simulink model "MCSI_simulation_2024_final_sim"  (R2021a)
settings: Solver=VariableStepAuto  StartTime=0.0  StopTime=10/cfg.fl  RelTol=1e-3
undefined symbols (not defined in the file or in its folder): cfg
libraries: spsIdealSwitchLib x18, simulink x17, hdlsllib x12, spsSeriesRLCBranchLib x8, spsCurrentMeasurementLib x6, commutil2 x6, spsMosfetLib x4, spsTriangleGeneratorLib x3, spsThreePhaseProgrammableGeneratorLib x3, spsMeanLib x2, spsThreePhaseSeriesRLCBranchLib x2, spsThreePhaseVIMeasurementLib x2
(part 1 of 2)
settings Model: Creator=Damian  LastModifiedBy=Damian

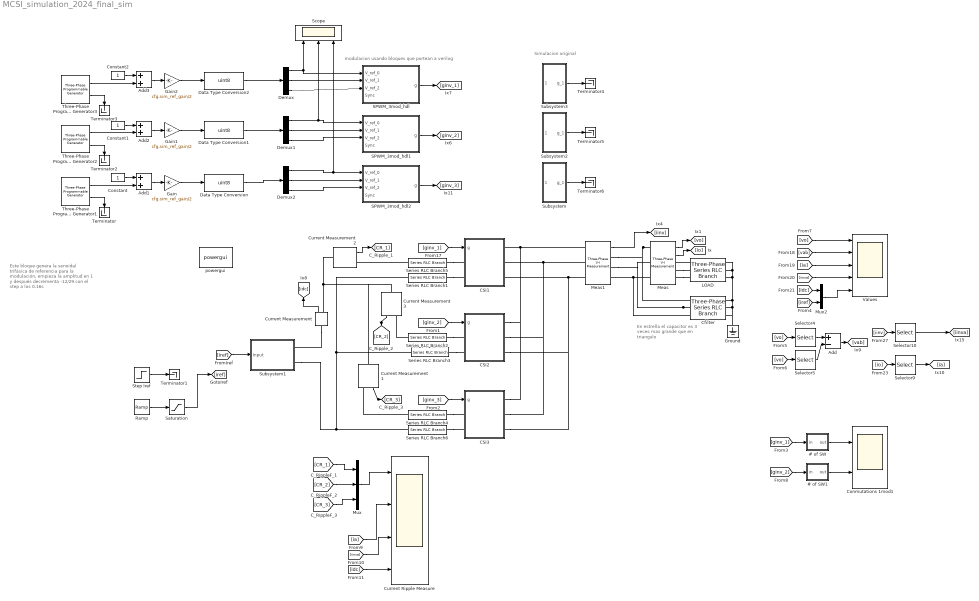
== system MCSI_simulation_2024_final_sim ==
  note: modulacion usando bloques que portean a verilog
  note: Simulacion original
  note: Este bloque genera la senoidal
      | trifásica de referencia para la
      | modulación, empieza la amplitud
      | en 1 y después decrementa -12/29
      | con el step a los 0.16s
  note: En estrella el capacitor
      | es 3 veces mas grande
      | que en triangulo
  # of SW : Subsystem
  # of SW1 : Subsystem
  Add : Sum  Inputs=+-
  Add1 : Sum
  Add2 : Sum
  Add3 : Sum
  CSI1 : Subsystem
  CSI2 : Subsystem
  CSI3 : Subsystem
  Cfilter : spsThreePhaseSeriesRLCBranchLib/Three-Phase Series RLC Branch  LConnTagsString=A|B|C  RConnTagsString=A|B|C  BranchType=C  Resistance=1  Inductance=cfg.c  Capacitance=cfg.c  Measurements=None
  Conmutations 1mod1 : Scope  NumInputPorts=2
  Constant : Constant
  Constant1 : Constant
  Constant2 : Constant
  Current Measurement{,1..3} (4 alike) : spsCurrentMeasurementLib/Current Measurement  PhasorSimulation=off  OutputType=Complex  PSBequivalent=0
  Current Ripple Measure : Scope  NumInputPorts=4
  Data Type Conversion : DataTypeConversion  OutDataTypeStr=uint8
  Data Type Conversion1 : DataTypeConversion  OutDataTypeStr=uint8
  Data Type Conversion2 : DataTypeConversion  OutDataTypeStr=uint8
  Demux : Demux  Outputs=3
  Demux1 : Demux  Outputs=3
  Demux2 : Demux  Outputs=3
  Gain : Gain  Gain=cfg.sim_ref_gain/2
  Gain1 : Gain  Gain=cfg.sim_ref_gain/2
  Gain2 : Gain  Gain=cfg.sim_ref_gain/2
  Ground : spsGroundLib/Ground  LConnTagsString=a
  LOAD : spsThreePhaseSeriesRLCBranchLib/Three-Phase Series RLC Branch  LConnTagsString=A|B|C  RConnTagsString=A|B|C  BranchType=RL  Resistance=cfg.r  Inductance=cfg.l  Capacitance=1e-6  Measurements=None
  Meas : spsThreePhaseVIMeasurementLib/Three-Phase V-I Measurement  VoltageMeasurement=phase-to-ground  SetLabelV=off  LabelV=Vabc  Vpu=off  VpuLL=off  CurrentMeasurement=yes  SetLabelI=off  LabelI=Iabc  Ipu=off  Pbase=100e6  Vbase=500e3  OutputType=Complex  PhasorSimulation=off  PSBequivalent=0
  Meas1 : spsThreePhaseVIMeasurementLib/Three-Phase V-I Measurement  VoltageMeasurement=no  SetLabelV=off  LabelV=Vabc  Vpu=off  VpuLL=off  CurrentMeasurement=yes  SetLabelI=off  LabelI=Iabc  Ipu=off  Pbase=100e6  Vbase=500e3  OutputType=Complex  PhasorSimulation=off  PSBequivalent=0
  Mux : Mux  Inputs=3
  Mux2 : Mux  Inputs=2
  Ramp : simulink/Sources/Ramp  slope=cfg.iref/cfg.cs_soft_start_time  start=0  InitialOutput=0
  SPWM_3mod_hdl : Subsystem
  SPWM_3mod_hdl1 : Subsystem
  SPWM_3mod_hdl2 : Subsystem
  Saturation : Saturate  UpperLimit=cfg.iref  LowerLimit=0
  Scope : Scope  NumInputPorts=3
  Selector10 : Selector  InputPortWidth=3  IndexOptions=Index vector (dialog)  Indices=1  OutputSizes=1
  Selector4 : Selector  InputPortWidth=3  IndexOptions=Index vector (dialog)  Indices=1  OutputSizes=1
  Selector5 : Selector  InputPortWidth=3  IndexOptions=Index vector (dialog)  Indices=2  OutputSizes=1
  Selector9 : Selector  InputPortWidth=3  IndexOptions=Index vector (dialog)  Indices=1  OutputSizes=1
  Series RLC Branch1 : spsSeriesRLCBranchLib/Series RLC Branch  LConnTagsString=__new0  RConnTagsString=__new0  BranchType=RL  Resistance=cfg.sharing_R  Inductance=cfg.sharing_L-0.16*cfg.sharing_L  SetiL0=off  InitialCurrent=0  Capacitance=1e-6  Setx0=off  InitialVoltage=0  Measurements=None
  Series RLC Branch2 : spsSeriesRLCBranchLib/Series RLC Branch  LConnTagsString=__new0  RConnTagsString=__new0  BranchType=RL  Resistance=cfg.sharing_R  Inductance=cfg.sharing_L  SetiL0=off  InitialCurrent=0  Capacitance=1e-6  Setx0=off  InitialVoltage=0  Measurements=None
  Series RLC Branch3 : spsSeriesRLCBranchLib/Series RLC Branch  LConnTagsString=__new0  RConnTagsString=__new0  BranchType=RL  Resistance=cfg.sharing_R  Inductance=cfg.sharing_L-0.2*cfg.sharing_L  SetiL0=off  InitialCurrent=0  Capacitance=1e-6  Setx0=off  InitialVoltage=0  Measurements=None
  Series RLC Branch4 : spsSeriesRLCBranchLib/Series RLC Branch  LConnTagsString=__new0  RConnTagsString=__new0  BranchType=RL  Resistance=cfg.sharing_R  Inductance=cfg.sharing_L-0.1*cfg.sharing_L  SetiL0=off  InitialCurrent=0  Capacitance=1e-6  Setx0=off  InitialVoltage=0  Measurements=None
  Series RLC Branch5 : spsSeriesRLCBranchLib/Series RLC Branch  LConnTagsString=__new0  RConnTagsString=__new0  BranchType=RL  Resistance=cfg.sharing_R  Inductance=cfg.sharing_L+0.2*cfg.sharing_L  SetiL0=off  InitialCurrent=0  Capacitance=1e-6  Setx0=off  InitialVoltage=0  Measurements=None
  Series RLC Branch6 : spsSeriesRLCBranchLib/Series RLC Branch  LConnTagsString=__new0  RConnTagsString=__new0  BranchType=RL  Resistance=cfg.sharing_R  Inductance=cfg.sharing_L+0.1*cfg.sharing_L  SetiL0=off  InitialCurrent=0  Capacitance=1e-6  Setx0=off  InitialVoltage=0  Measurements=None
  Step Iref : Step  Time=12/cfg.fl  Before=cfg.iref  After=0.6*cfg.iref  SampleTime=cfg.ts
  Subsystem : Subsystem
  Subsystem1 : Subsystem
  Subsystem2 : Subsystem
  Subsystem3 : Subsystem
  Terminator{,1..6} (7 alike) : Terminator
  Three-Phase Programmable Generator1 : spsThreePhaseProgrammableGeneratorLib/Three-Phase Programmable Generator  Par_Vps=[0.9999,0, cfg.fl]  VariationEntity=None  VariationType=Step  VariationStep=-12/29  VariationRate=10  VariationMag=0.3  VariationFreq=2  Par_Timing_Variation="[8/cfg.fl  10]"  SinglePhase=on  Yampli=[1 0.2 1.2 1.0]  Xtime=[0 0.1 0.15 0.2]  HarmonicGeneration=off  Par_HarmoA="[3  5  -25 0]"  Par_HarmoB="[5  10  35  2]"  Par_Timing_Harmo="[ 0.05  99]"  Ts=cfg.ts*100
      settings: SourceProductBaseCode=PS
  Three-Phase Programmable Generator2 : spsThreePhaseProgrammableGeneratorLib/Three-Phase Programmable Generator  Par_Vps=[0.9999,0, cfg.fl]  VariationEntity=None  VariationType=Step  VariationStep=-12/29  VariationRate=10  VariationMag=0.3  VariationFreq=2  Par_Timing_Variation="[8/cfg.fl  10]"  SinglePhase=on  Yampli=[1 0.2 1.2 1.0]  Xtime=[0 0.1 0.15 0.2]  HarmonicGeneration=off  Par_HarmoA="[3  5  -25 0]"  Par_HarmoB="[5  10  35  2]"  Par_Timing_Harmo="[ 0.05  99]"  Ts=cfg.ts*100
      settings: SourceProductBaseCode=PS
  Three-Phase Programmable Generator3 : spsThreePhaseProgrammableGeneratorLib/Three-Phase Programmable Generator  Par_Vps=[0.9999,0, cfg.fl]  VariationEntity=None  VariationType=Step  VariationStep=-12/29  VariationRate=10  VariationMag=0.3  VariationFreq=2  Par_Timing_Variation="[8/cfg.fl  10]"  SinglePhase=on  Yampli=[1 0.2 1.2 1.0]  Xtime=[0 0.1 0.15 0.2]  HarmonicGeneration=off  Par_HarmoA="[3  5  -25 0]"  Par_HarmoB="[5  10  35  2]"  Par_Timing_Harmo="[ 0.05  99]"  Ts=cfg.ts*100
      settings: SourceProductBaseCode=PS
  Values : Scope  NumInputPorts=5
  powergui : spspowerguiLib/powergui  Priority=1  SimulationMode=Discrete  SampleTime=cfg.ts  frequency=60  Iterations=50  frequencyindice=0  Pbase=100e6  ErrMax=1e-4  UnitsV=kV  UnitsW=MW  buscounter=0  FunctionMessages=off  echomessages=off  EnableUseOfTLC=off  CurrentSourceSwitches=off  DisableSnubberDevices=off  DisableRonSwitches=off  DisableVfSwitches=off  DisplayEquations=off  AutomaticDiscreteSolvers=off  SolverType=Backward Euler  Interpol=off  ExternalGateDelay=off  methode=off  Ts=0  x0status=blocks  SPID=off  SwTol=0  HookPort=off  NonlinearTolerance=1e-4  nMaxIteration=100  ContinueOnMaxIteration=off  RestoreLinks=warning  ResistiveCurrentMeasurement=off  Frange=[0:2:500]  Ylog=off  Xlog=on  ShowGrid=off  save=off  variable=ZData  structure=one_mod_model  ZoomFFT=off  StartTime=0.12  cycles=1  DisplayStyle=1  fundamental=50  FreqAxis=off  MaxFrequency=1000  frequencyindicesteady=1  RmsSteady=1  display=off
  wires:
  Current Measurement/1 -> [idc]
  Three-Phase Programmable Generator1/2 -> Terminator/1
  [ginv_1] -> CSI1/1(g)
  Meas/1 -> [vo]
  Meas/2 -> [io]
  Meas1/1 -> [iinv]
  [iref] -> Mux2/2
  [idc] -> Mux2/1
  Mux2/1 -> Values/5
  [vo] -> Values/1
  [iinva] -> Values/4
  [ia] -> Values/3
  [vab] -> Values/2
  [vo] -> Selector4/1
  [vo] -> Selector5/1
  Selector4/1 -> Add/1
  Selector5/1 -> Add/2
  Add/1 -> [vab]
  [iinv] -> Selector10/1
  [io] -> Selector9/1
  Selector10/1 -> [iinva]
  Selector9/1 -> [ia]
  [ginv_2] -> CSI2/1(g)
  [ginv_3] -> CSI3/1(g)
  [ginv_1] -> # of SW/1(in)
  # of SW/1(out) -> Conmutations 1mod1/1
  # of SW1/1(out) -> Conmutations 1mod1/2
  [ginv_2] -> # of SW1/1(in)
  Saturation/1 -> [iref]
  Ramp/1 -> Saturation/1
  Step Iref/1 -> Terminator1/1
  Current Measurement2/1 -> [CR_1]
  Current Measurement3/1 -> [CR_2]
  Current Measurement1/1 -> [CR_3]
  [ia] -> Current Ripple Measure/2
  [iinva] -> Current Ripple Measure/3
  [idc] -> Current Ripple Measure/4
  [CR_1] -> Mux/1
  [CR_2] -> Mux/2
  [CR_3] -> Mux/3
  Mux/1 -> Current Ripple Measure/1
  [iref] -> Subsystem1/1(Input)
  Constant/1 -> Add1/1
  Gain/1 -> Data Type Conversion/1
  Add1/1 -> Gain/1
  Three-Phase Programmable Generator1/1 -> Add1/2
  Add2/1 -> Gain1/1
  Gain1/1 -> Data Type Conversion1/1
  Constant1/1 -> Add2/1
  Three-Phase Programmable Generator2/2 -> Terminator2/1
  Add3/1 -> Gain2/1
  Gain2/1 -> Data Type Conversion2/1
  Constant2/1 -> Add3/1
  Three-Phase Programmable Generator3/2 -> Terminator3/1
  Three-Phase Programmable Generator3/1 -> Add3/2
  Three-Phase Programmable Generator2/1 -> Add2/2
  Data Type Conversion2/1 -> Demux/1
  SPWM_3mod_hdl/1(g) -> [ginv_1]
  SPWM_3mod_hdl1/1(g) -> [ginv_2]
  SPWM_3mod_hdl2/1(g) -> [ginv_3]
  Demux/3 -> SPWM_3mod_hdl/3(V_ref_2)
  Demux/2 -> SPWM_3mod_hdl/2(V_ref_1)
  Demux/1 -> Scope/1, SPWM_3mod_hdl/1(V_ref_0)
  Demux1/3 -> SPWM_3mod_hdl1/3(V_ref_2)
  Demux1/2 -> SPWM_3mod_hdl1/2(V_ref_1)
  Demux1/1 -> Scope/2, SPWM_3mod_hdl1/1(V_ref_0)
  Demux2/3 -> SPWM_3mod_hdl2/3(V_ref_2)
  Demux2/2 -> SPWM_3mod_hdl2/2(V_ref_1)
  Demux2/1 -> SPWM_3mod_hdl2/1(V_ref_0), Scope/3
  Data Type Conversion/1 -> Demux2/1
  Data Type Conversion1/1 -> Demux1/1
  Subsystem/1(g_1) -> Terminator6/1
  Subsystem3/1(g_1) -> Terminator4/1
  Subsystem2/1(g_1) -> Terminator5/1
  connections:
  Current Measurement/LConn1 -- Subsystem1/RConn1
  Meas/LConn3 -- Cfilter/LConn3 -- Meas1/RConn3
  Meas/LConn1 -- Meas1/RConn1 -- Cfilter/LConn1
  LOAD/RConn2 -- LOAD/RConn1 -- LOAD/RConn3 -- Cfilter/RConn1 -- Cfilter/RConn2 -- Cfilter/RConn3 -- Ground/LConn1
  Cfilter/LConn2 -- Meas1/RConn2 -- Meas/LConn2
  LOAD/LConn1 -- Meas/RConn1
  Meas/RConn2 -- LOAD/LConn2
  Meas/RConn3 -- LOAD/LConn3
  Meas1/LConn1 -- CSI3/RConn1 -- CSI2/RConn1 -- CSI1/RConn1
  Meas1/LConn2 -- CSI3/RConn2 -- CSI2/RConn2 -- CSI1/RConn2
  Meas1/LConn3 -- CSI3/RConn3 -- CSI2/RConn3 -- CSI1/RConn3
  Series RLC Branch1/RConn1 -- CSI1/LConn2
  Series RLC Branch5/RConn1 -- CSI1/LConn1
  Series RLC Branch2/RConn1 -- CSI2/LConn1
  Series RLC Branch3/RConn1 -- CSI2/LConn2
  Series RLC Branch4/RConn1 -- CSI3/LConn1
  Series RLC Branch6/RConn1 -- CSI3/LConn2
  Subsystem1/RConn2 -- Series RLC Branch6/LConn1 -- Series RLC Branch3/LConn1 -- Series RLC Branch1/LConn1
  Series RLC Branch2/LConn1 -- Current Measurement3/RConn1
  Current Measurement2/LConn1 -- Current Measurement3/LConn1 -- Current Measurement1/LConn1 -- Current Measurement/RConn1
  Series RLC Branch4/LConn1 -- Current Measurement1/RConn1
  Series RLC Branch5/LConn1 -- Current Measurement2/RConn1

== system MCSI_simulation_2024_final_sim/# of SW ==
  in : Inport
  Data Type Conversion : DataTypeConversion
  Detect Change : simulink/Logic and Bit Operations/Detect Change  vinit=0  OutDataTypeStr=boolean
  Divide : Product  Inputs=*/
  Gain : Gain  Gain=1/cfg.ts
  Mean1 : spsMeanLib/Mean  Freq=cfg.fl  Vinit=0  Ts=cfg.ts
  Sum of Elements : Sum  Inputs=+
  Width : Width
  out : Outport
  wires:
  Detect Change/1 -> Data Type Conversion/1
  Mean1/1 -> Gain/1
  Data Type Conversion/1 -> Mean1/1
  in/1 -> Detect Change/1
  Gain/1 -> Width/1, Sum of Elements/1
  Sum of Elements/1 -> Divide/1
  Width/1 -> Divide/2
  Divide/1 -> out/1

== system MCSI_simulation_2024_final_sim/# of SW1 ==
  in : Inport
  Data Type Conversion : DataTypeConversion
  Detect Change : simulink/Logic and Bit Operations/Detect Change  vinit=0  OutDataTypeStr=boolean
  Gain : Gain  Gain=1/cfg.ts
  Mean1 : spsMeanLib/Mean  Freq=cfg.fl  Vinit=0  Ts=cfg.ts
  out : Outport
  wires:
  Detect Change/1 -> Data Type Conversion/1
  Mean1/1 -> Gain/1
  Data Type Conversion/1 -> Mean1/1
  in/1 -> Detect Change/1
  Gain/1 -> out/1

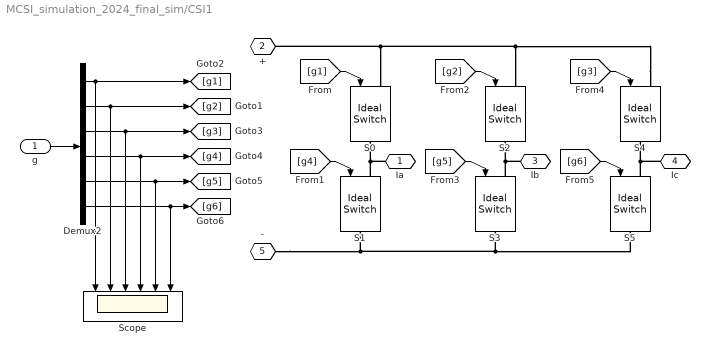
== system MCSI_simulation_2024_final_sim/CSI1 ==
  g : Inport
  Demux2 : Demux  Outputs=6
  S{0..5} (6 alike) : spsIdealSwitchLib/Ideal Switch  Ron=cfg.switch.Ron  Lon=0  IC=0  Rs=cfg.switch.snubber_Rs  Cs=cfg.switch.snubber_Cs  Measurements=off
  Scope : Scope  NumInputPorts=6
  Ia : PMIOPort  Side=Right
  + : PMIOPort  Port=2  Side=Left
  Ib : PMIOPort  Port=3  Side=Right
  Ic : PMIOPort  Port=4  Side=Right
  - : PMIOPort  Port=5  Side=Left
  wires:
  Demux2/1 -> [g1], Scope/1
  Demux2/4 -> [g4], Scope/4
  g/1 -> Demux2/1
  [g4] -> S1/1
  [g2] -> S2/1
  [g5] -> S3/1
  Demux2/5 -> [g5], Scope/5
  [g3] -> S4/1
  [g6] -> S5/1
  Demux2/6 -> Scope/6, [g6]
  Demux2/3 -> Scope/3, [g3]
  Demux2/2 -> Scope/2, [g2]
  [g1] -> S0/1
  connections:
  S1/LConn1 -- Ia/RConn1 -- S0/RConn1
  S3/LConn1 -- Ib/RConn1 -- S2/RConn1
  S5/LConn1 -- Ic/RConn1 -- S4/RConn1
  S4/LConn1 -- S2/LConn1 -- S0/LConn1 -- +/RConn1
  -/RConn1 -- S5/RConn1 -- S3/RConn1 -- S1/RConn1

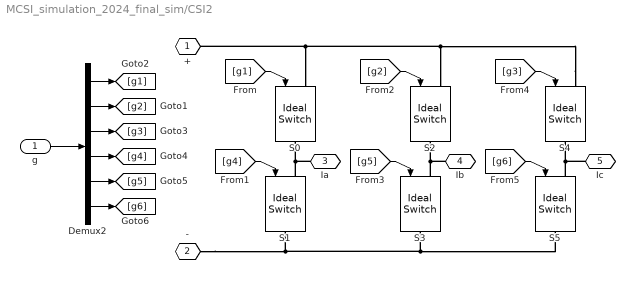
== system MCSI_simulation_2024_final_sim/CSI2 ==
  g : Inport
  Demux2 : Demux  Outputs=6
  S{0..5} (6 alike) : spsIdealSwitchLib/Ideal Switch  Ron=cfg.switch.Ron  Lon=0  IC=0  Rs=cfg.switch.snubber_Rs  Cs=cfg.switch.snubber_Cs  Measurements=off
  + : PMIOPort  Side=Left
  - : PMIOPort  Port=2  Side=Left
  Ia : PMIOPort  Port=3  Side=Right
  Ib : PMIOPort  Port=4  Side=Right
  Ic : PMIOPort  Port=5  Side=Right
  wires:
  Demux2/1 -> [g1]
  Demux2/4 -> [g4]
  g/1 -> Demux2/1
  [g4] -> S1/1
  [g2] -> S2/1
  [g5] -> S3/1
  Demux2/5 -> [g5]
  [g3] -> S4/1
  [g6] -> S5/1
  Demux2/6 -> [g6]
  Demux2/3 -> [g3]
  Demux2/2 -> [g2]
  [g1] -> S0/1
  connections:
  S1/LConn1 -- Ia/RConn1 -- S0/RConn1
  S3/LConn1 -- Ib/RConn1 -- S2/RConn1
  S5/LConn1 -- Ic/RConn1 -- S4/RConn1
  S4/LConn1 -- S2/LConn1 -- S0/LConn1 -- +/RConn1
  -/RConn1 -- S5/RConn1 -- S3/RConn1 -- S1/RConn1

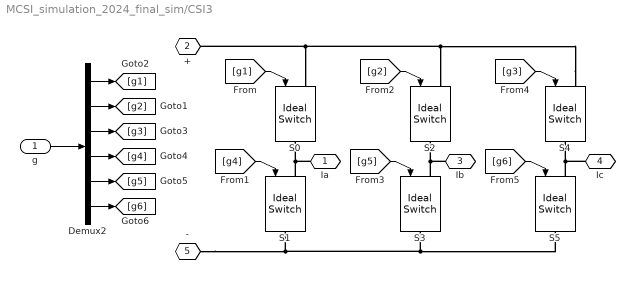
== system MCSI_simulation_2024_final_sim/CSI3 ==
  g : Inport
  Demux2 : Demux  Outputs=6
  S{0..5} (6 alike) : spsIdealSwitchLib/Ideal Switch  Ron=cfg.switch.Ron  Lon=0  IC=0  Rs=cfg.switch.snubber_Rs  Cs=cfg.switch.snubber_Cs  Measurements=off
  Ia : PMIOPort  Side=Right
  + : PMIOPort  Port=2  Side=Left
  Ib : PMIOPort  Port=3  Side=Right
  Ic : PMIOPort  Port=4  Side=Right
  - : PMIOPort  Port=5  Side=Left
  wires:
  Demux2/1 -> [g1]
  Demux2/4 -> [g4]
  g/1 -> Demux2/1
  [g4] -> S1/1
  [g2] -> S2/1
  [g5] -> S3/1
  Demux2/5 -> [g5]
  [g3] -> S4/1
  [g6] -> S5/1
  Demux2/6 -> [g6]
  Demux2/3 -> [g3]
  Demux2/2 -> [g2]
  [g1] -> S0/1
  connections:
  S1/LConn1 -- Ia/RConn1 -- S0/RConn1
  S3/LConn1 -- Ib/RConn1 -- S2/RConn1
  S5/LConn1 -- Ic/RConn1 -- S4/RConn1
  S4/LConn1 -- S2/LConn1 -- S0/LConn1 -- +/RConn1
  -/RConn1 -- S5/RConn1 -- S3/RConn1 -- S1/RConn1

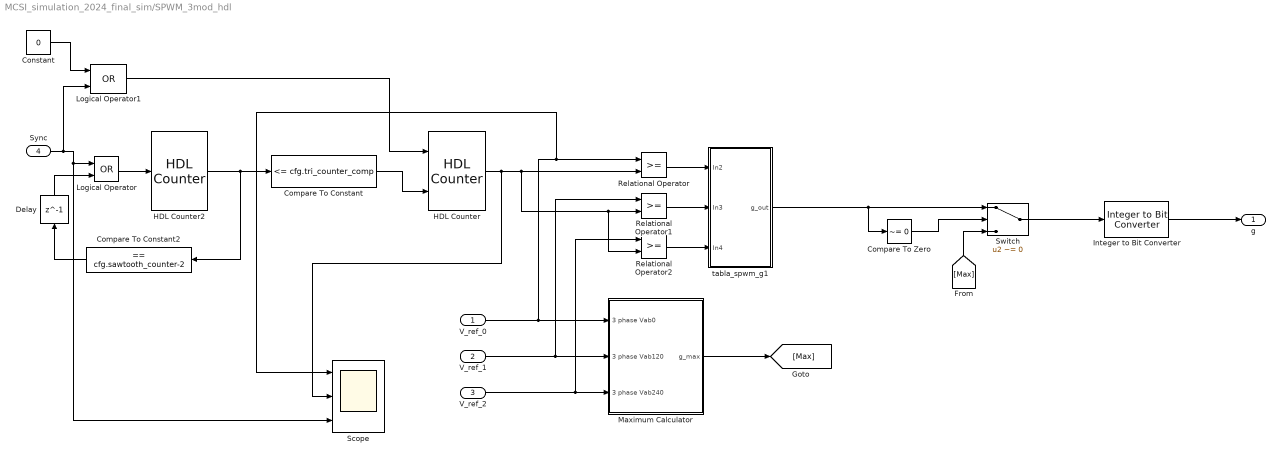
== system MCSI_simulation_2024_final_sim/SPWM_3mod_hdl ==
  V_ref_0 : Inport  OutDataTypeStr=fixdt(0,8,0)
  V_ref_1 : Inport  Port=2  OutDataTypeStr=fixdt(0,8,0)
  V_ref_2 : Inport  Port=3  OutDataTypeStr=fixdt(0,8,0)
  Sync : Inport  Port=4
  Compare To Constant : simulink/Logic and Bit Operations/Compare To Constant  relop=<=  const=cfg.tri_counter_comp  OutDataTypeStr=boolean
  Compare To Constant2 : simulink/Logic and Bit Operations/Compare To Constant  relop===  const=cfg.sawtooth_counter-2  OutDataTypeStr=boolean
  Compare To Zero : simulink/Logic and Bit Operations/Compare To Zero  relop=~=  OutDataTypeStr=boolean
  Constant : Constant  Value=0
  Delay : Delay  DelayLength=1  InitialCondition=0
  HDL Counter : hdlsllib/Sources/HDL Counter  CountType=Free running  CountInit=0  CountStep=1  CountMax=255  CountFromType=Initial value  CountFrom=0  CountResetPort=on  CountLoadPort=off  CountEnbPort=off  CountDirPort=on  CountHitOutputPort=off  CountDataType=Unsigned  CountWordLen=cfg.counter_tri_word_length  CountFracLen=0  CountSampTime=1
  HDL Counter2 : hdlsllib/Sources/HDL Counter  CountType=Free running  CountInit=0  CountStep=1  CountMax=cfg.sawtooth_counter-1  CountFromType=Initial value  CountFrom=0  CountResetPort=on  CountLoadPort=off  CountEnbPort=off  CountDirPort=off  CountHitOutputPort=off  CountDataType=Unsigned  CountWordLen=cfg.counter_word_length  CountFracLen=0  CountSampTime=1
  Integer to Bit Converter : commutil2/Integer to Bit Converter  nbits=6  signedInputValues=Unsigned  bitOrder=MSB first  outDtype=Inherit via internal rule
  Logical Operator : Logic  Operator=OR  AllPortsSameDT=off  OutDataTypeStr=boolean
  Logical Operator1 : Logic  Operator=OR  AllPortsSameDT=off  OutDataTypeStr=boolean
  Maximum Calculator : Subsystem
  Relational Operator : RelationalOperator  OutDataTypeStr=boolean  RndMeth=Nearest
  Relational Operator1 : RelationalOperator  OutDataTypeStr=boolean  RndMeth=Nearest
  Relational Operator2 : RelationalOperator  OutDataTypeStr=boolean  RndMeth=Nearest
  Scope : Scope  NumInputPorts=3
  Switch : Switch  Criteria=u2 ~= 0
  tabla_spwm_g1 : Subsystem
  g : Outport
  wires:
  V_ref_2/1 -> Maximum Calculator/3(3 phase Vab240), Relational Operator2/1
  [Max] -> Switch/3
  Relational Operator1/1 -> tabla_spwm_g1/2(In3)
  tabla_spwm_g1/1(g_out) -> Compare To Zero/1, Switch/1
  Relational Operator/1 -> tabla_spwm_g1/1(In2)
  V_ref_1/1 -> Maximum Calculator/2(3 phase Vab120), Relational Operator1/1
  V_ref_0/1 -> Maximum Calculator/1(3 phase Vab0), Scope/1, Relational Operator/1
  Compare To Constant2/1 -> Delay/1
  Maximum Calculator/1(g_max) -> [Max]
  HDL Counter/1 -> Scope/2, Relational Operator2/2, Relational Operator1/2, Relational Operator/2
  Compare To Zero/1 -> Switch/2
  Relational Operator2/1 -> tabla_spwm_g1/3(In4)
  Compare To Constant/1 -> HDL Counter/2
  HDL Counter2/1 -> Compare To Constant/1, Compare To Constant2/1
  Logical Operator/1 -> HDL Counter2/1
  Delay/1 -> Logical Operator/2
  Sync/1 -> Logical Operator1/2, Scope/3, Logical Operator/1
  Logical Operator1/1 -> HDL Counter/1
  Constant/1 -> Logical Operator1/1
  Integer to Bit Converter/1 -> g/1
  Switch/1 -> Integer to Bit Converter/1

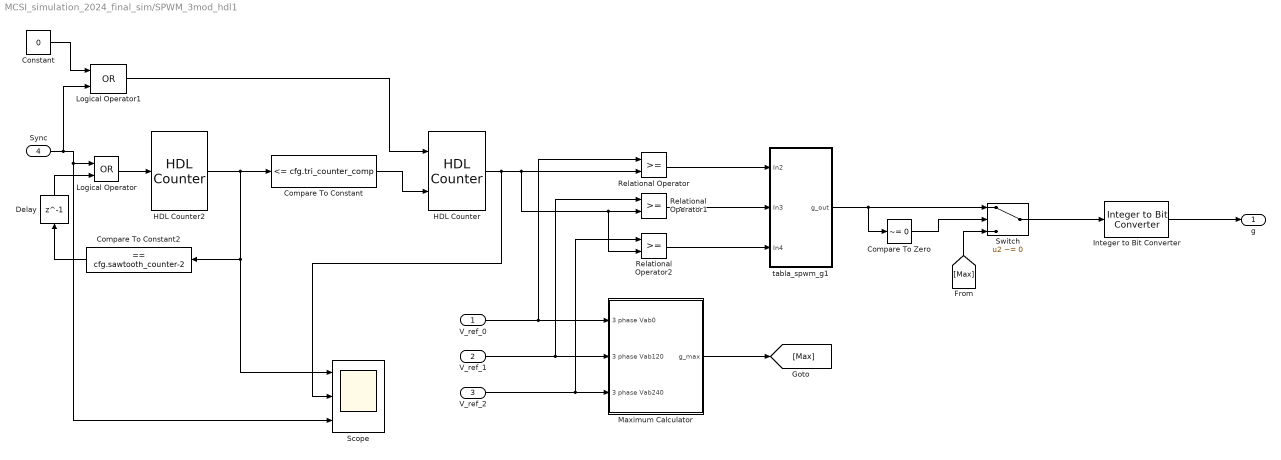
== system MCSI_simulation_2024_final_sim/SPWM_3mod_hdl1 ==
  V_ref_0 : Inport  OutDataTypeStr=fixdt(0,8,0)
  V_ref_1 : Inport  Port=2  OutDataTypeStr=fixdt(0,8,0)
  V_ref_2 : Inport  Port=3  OutDataTypeStr=fixdt(0,8,0)
  Sync : Inport  Port=4
  Compare To Constant : simulink/Logic and Bit Operations/Compare To Constant  relop=<=  const=cfg.tri_counter_comp  OutDataTypeStr=boolean
  Compare To Constant2 : simulink/Logic and Bit Operations/Compare To Constant  relop===  const=cfg.sawtooth_counter-2  OutDataTypeStr=boolean
  Compare To Zero : simulink/Logic and Bit Operations/Compare To Zero  relop=~=  OutDataTypeStr=boolean
  Constant : Constant  Value=0
  Delay : Delay  DelayLength=1  InitialCondition=0
  HDL Counter : hdlsllib/Sources/HDL Counter  CountType=Free running  CountInit=0  CountStep=1  CountMax=255  CountFromType=Initial value  CountFrom=0  CountResetPort=on  CountLoadPort=off  CountEnbPort=off  CountDirPort=on  CountHitOutputPort=off  CountDataType=Unsigned  CountWordLen=cfg.counter_tri_word_length  CountFracLen=0  CountSampTime=1
  HDL Counter2 : hdlsllib/Sources/HDL Counter  CountType=Free running  CountInit=0  CountStep=1  CountMax=cfg.sawtooth_counter-1  CountFromType=Initial value  CountFrom=0  CountResetPort=on  CountLoadPort=off  CountEnbPort=off  CountDirPort=off  CountHitOutputPort=off  CountDataType=Unsigned  CountWordLen=cfg.counter_word_length  CountFracLen=0  CountSampTime=1
  Integer to Bit Converter : commutil2/Integer to Bit Converter  nbits=6  signedInputValues=Unsigned  bitOrder=MSB first  outDtype=Inherit via internal rule
  Logical Operator : Logic  Operator=OR  AllPortsSameDT=off  OutDataTypeStr=boolean
  Logical Operator1 : Logic  Operator=OR  AllPortsSameDT=off  OutDataTypeStr=boolean
  Maximum Calculator : Subsystem
  Relational Operator : RelationalOperator  OutDataTypeStr=boolean  RndMeth=Nearest
  Relational Operator1 : RelationalOperator  OutDataTypeStr=boolean  RndMeth=Nearest
  Relational Operator2 : RelationalOperator  OutDataTypeStr=boolean  RndMeth=Nearest
  Scope : Scope  NumInputPorts=3
  Switch : Switch  Criteria=u2 ~= 0
  tabla_spwm_g1 : Subsystem
  g : Outport
  wires:
  V_ref_2/1 -> Maximum Calculator/3(3 phase Vab240), Relational Operator2/1
  [Max] -> Switch/3
  Relational Operator1/1 -> tabla_spwm_g1/2(In3)
  tabla_spwm_g1/1(g_out) -> Compare To Zero/1, Switch/1
  Relational Operator/1 -> tabla_spwm_g1/1(In2)
  V_ref_1/1 -> Maximum Calculator/2(3 phase Vab120), Relational Operator1/1
  V_ref_0/1 -> Maximum Calculator/1(3 phase Vab0), Relational Operator/1
  Compare To Constant2/1 -> Delay/1
  Maximum Calculator/1(g_max) -> [Max]
  HDL Counter/1 -> Scope/2, Relational Operator2/2, Relational Operator1/2, Relational Operator/2
  Compare To Zero/1 -> Switch/2
  Relational Operator2/1 -> tabla_spwm_g1/3(In4)
  Compare To Constant/1 -> HDL Counter/2
  HDL Counter2/1 -> Compare To Constant/1, Scope/1, Compare To Constant2/1
  Logical Operator/1 -> HDL Counter2/1
  Delay/1 -> Logical Operator/2
  Sync/1 -> Logical Operator1/2, Scope/3, Logical Operator/1
  Logical Operator1/1 -> HDL Counter/1
  Constant/1 -> Logical Operator1/1
  Integer to Bit Converter/1 -> g/1
  Switch/1 -> Integer to Bit Converter/1

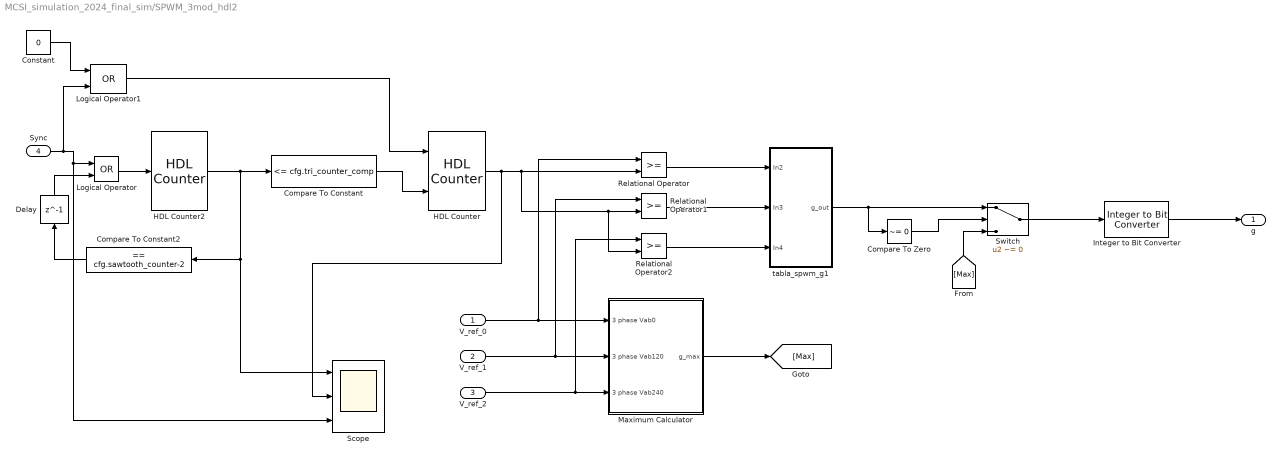
== system MCSI_simulation_2024_final_sim/SPWM_3mod_hdl2 ==
  V_ref_0 : Inport  OutDataTypeStr=fixdt(0,8,0)
  V_ref_1 : Inport  Port=2  OutDataTypeStr=fixdt(0,8,0)
  V_ref_2 : Inport  Port=3  OutDataTypeStr=fixdt(0,8,0)
  Sync : Inport  Port=4
  Compare To Constant : simulink/Logic and Bit Operations/Compare To Constant  relop=<=  const=cfg.tri_counter_comp  OutDataTypeStr=boolean
  Compare To Constant2 : simulink/Logic and Bit Operations/Compare To Constant  relop===  const=cfg.sawtooth_counter-2  OutDataTypeStr=boolean
  Compare To Zero : simulink/Logic and Bit Operations/Compare To Zero  relop=~=  OutDataTypeStr=boolean
  Constant : Constant  Value=0
  Delay : Delay  DelayLength=1  InitialCondition=0
  HDL Counter : hdlsllib/Sources/HDL Counter  CountType=Free running  CountInit=0  CountStep=1  CountMax=255  CountFromType=Initial value  CountFrom=0  CountResetPort=on  CountLoadPort=off  CountEnbPort=off  CountDirPort=on  CountHitOutputPort=off  CountDataType=Unsigned  CountWordLen=cfg.counter_tri_word_length  CountFracLen=0  CountSampTime=1
  HDL Counter2 : hdlsllib/Sources/HDL Counter  CountType=Free running  CountInit=0  CountStep=1  CountMax=cfg.sawtooth_counter-1  CountFromType=Initial value  CountFrom=0  CountResetPort=on  CountLoadPort=off  CountEnbPort=off  CountDirPort=off  CountHitOutputPort=off  CountDataType=Unsigned  CountWordLen=cfg.counter_word_length  CountFracLen=0  CountSampTime=1
  Integer to Bit Converter : commutil2/Integer to Bit Converter  nbits=6  signedInputValues=Unsigned  bitOrder=MSB first  outDtype=Inherit via internal rule
  Logical Operator : Logic  Operator=OR  AllPortsSameDT=off  OutDataTypeStr=boolean
  Logical Operator1 : Logic  Operator=OR  AllPortsSameDT=off  OutDataTypeStr=boolean
  Maximum Calculator : Subsystem
  Relational Operator : RelationalOperator  OutDataTypeStr=boolean  RndMeth=Nearest
  Relational Operator1 : RelationalOperator  OutDataTypeStr=boolean  RndMeth=Nearest
  Relational Operator2 : RelationalOperator  OutDataTypeStr=boolean  RndMeth=Nearest
  Scope : Scope  NumInputPorts=3
  Switch : Switch  Criteria=u2 ~= 0
  tabla_spwm_g1 : Subsystem
  g : Outport
  wires:
  V_ref_2/1 -> Maximum Calculator/3(3 phase Vab240), Relational Operator2/1
  [Max] -> Switch/3
  Relational Operator1/1 -> tabla_spwm_g1/2(In3)
  tabla_spwm_g1/1(g_out) -> Compare To Zero/1, Switch/1
  Relational Operator/1 -> tabla_spwm_g1/1(In2)
  V_ref_1/1 -> Maximum Calculator/2(3 phase Vab120), Relational Operator1/1
  V_ref_0/1 -> Maximum Calculator/1(3 phase Vab0), Relational Operator/1
  Compare To Constant2/1 -> Delay/1
  Maximum Calculator/1(g_max) -> [Max]
  HDL Counter/1 -> Scope/2, Relational Operator2/2, Relational Operator1/2, Relational Operator/2
  Compare To Zero/1 -> Switch/2
  Relational Operator2/1 -> tabla_spwm_g1/3(In4)
  Compare To Constant/1 -> HDL Counter/2
  HDL Counter2/1 -> Compare To Constant/1, Scope/1, Compare To Constant2/1
  Logical Operator/1 -> HDL Counter2/1
  Delay/1 -> Logical Operator/2
  Sync/1 -> Logical Operator1/2, Scope/3, Logical Operator/1
  Logical Operator1/1 -> HDL Counter/1
  Constant/1 -> Logical Operator1/1
  Integer to Bit Converter/1 -> g/1
  Switch/1 -> Integer to Bit Converter/1

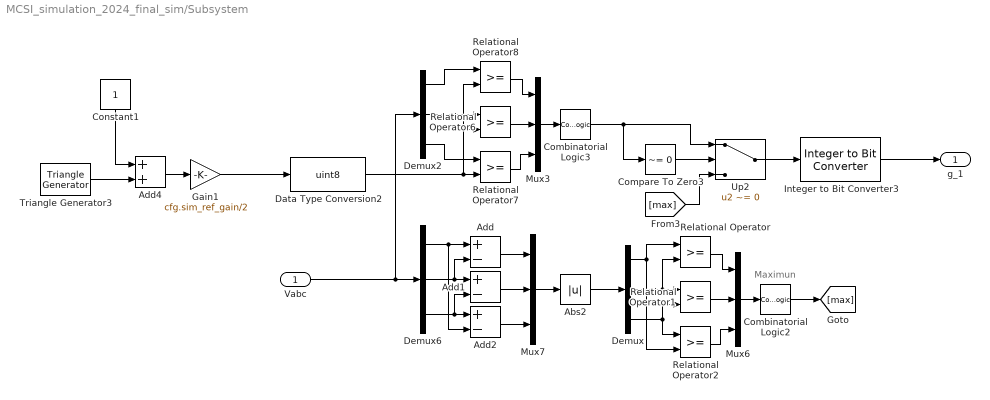
== system MCSI_simulation_2024_final_sim/Subsystem ==
  note: Maximun
  Vabc : Inport
  Abs2 : Abs
  Add : Sum  Inputs=+-
  Add1 : Sum  Inputs=+-
  Add2 : Sum  Inputs=+-
  Add4 : Sum
  Combinatorial Logic2 : CombinatorialLogic  TruthTable=bin2dec(['111111'; '001001'; '010010'; '010010'; '100100'; '001001'; '100100'; '111111'])
  Combinatorial Logic3 : CombinatorialLogic  TruthTable=bin2dec(['000000'; '001010'; '010100'; '001100'; '100001'; '100010'; '010001'; '000000'])
  Compare To Zero3 : simulink/Logic and Bit Operations/Compare To Zero  relop=~=  OutDataTypeStr=boolean
  Constant1 : Constant
  Data Type Conversion2 : DataTypeConversion  OutDataTypeStr=uint8
  Demux : Demux  Outputs=3
  Demux2 : Demux  Outputs=3
  Demux6 : Demux  Outputs=3
  Gain1 : Gain  Gain=cfg.sim_ref_gain/2
  Integer to Bit Converter3 : commutil2/Integer to Bit Converter  nbits=6  signedInputValues=Unsigned  bitOrder=MSB first  outDtype=Inherit via internal rule
  Mux3 : Mux  Inputs=3
  Mux6 : Mux  Inputs=3
  Mux7 : Mux  Inputs=3
  Relational Operator{,1..2,6..8} (6 alike) : RelationalOperator  OutDataTypeStr=boolean  RndMeth=Nearest
  Triangle Generator3 : spsTriangleGeneratorLib/Triangle Generator  Freq=cfg.fl*cfg.mf  Phase=0  Ts=cfg.ts
  Up2 : Switch  Criteria=u2 ~= 0
  g_1 : Outport
  wires:
  Relational Operator/1 -> Mux6/1
  Demux/3 -> Relational Operator1/2, Relational Operator2/1
  Relational Operator1/1 -> Mux6/2
  Demux/2 -> Relational Operator/2, Relational Operator1/1
  Mux6/1 -> Combinatorial Logic2/1
  Relational Operator2/1 -> Mux6/3
  Demux/1 -> Relational Operator/1, Relational Operator2/2
  Demux6/1 -> Add2/2, Add/1
  Demux6/2 -> Add/2, Add1/1
  Demux6/3 -> Add1/2, Add2/1
  Add/1 -> Mux7/1
  Add1/1 -> Mux7/2
  Add2/1 -> Mux7/3
  Abs2/1 -> Demux/1
  Mux7/1 -> Abs2/1
  Combinatorial Logic2/1 -> [max]
  Relational Operator7/1 -> Mux3/3
  Relational Operator8/1 -> Mux3/1
  Relational Operator6/1 -> Mux3/2
  Mux3/1 -> Combinatorial Logic3/1
  Combinatorial Logic3/1 -> Up2/1, Compare To Zero3/1
  Compare To Zero3/1 -> Up2/2
  Up2/1 -> Integer to Bit Converter3/1
  [max] -> Up2/3
  Demux2/3 -> Relational Operator7/1
  Demux2/2 -> Relational Operator6/1
  Demux2/1 -> Relational Operator8/1
  Integer to Bit Converter3/1 -> g_1/1
  Vabc/1 -> Demux2/1, Demux6/1
  Data Type Conversion2/1 -> Relational Operator8/2, Relational Operator6/2, Relational Operator7/2
  Gain1/1 -> Data Type Conversion2/1
  ? -> ?
  Constant1/1 -> Add4/1
  Triangle Generator3/1 -> Add4/2
  Add4/1 -> Gain1/1

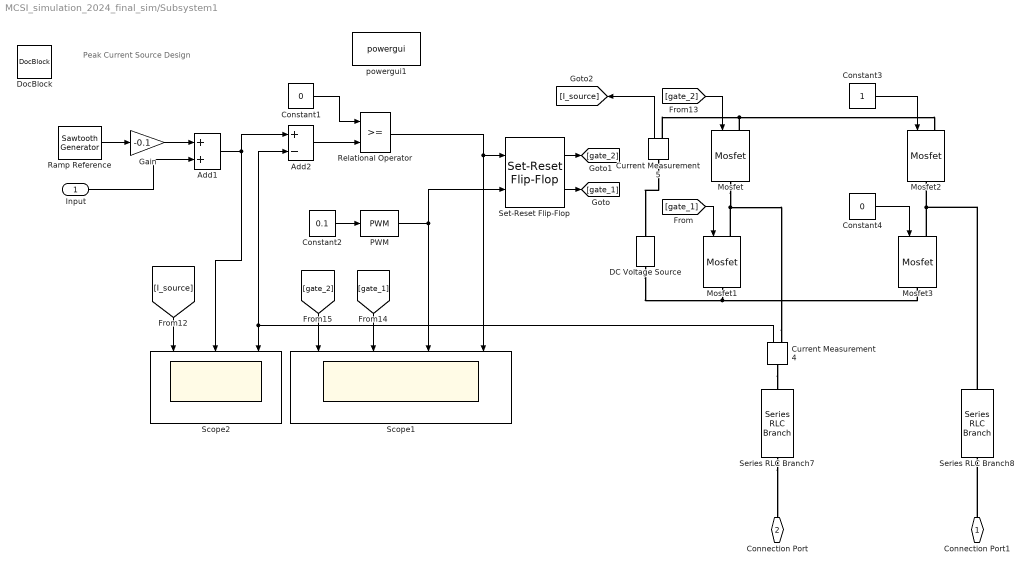
== system MCSI_simulation_2024_final_sim/Subsystem1 ==
  note: Peak Current Source Design
  Input : Inport
  Add1 : Sum
  Add2 : Sum  Inputs=+-
  Constant1 : Constant  Value=0
  Constant2 : Constant  Value=0.1
  Constant3 : Constant
  Constant4 : Constant  Value=0
  Current Measurement4 : spsCurrentMeasurementLib/Current Measurement  PhasorSimulation=off  OutputType=Complex  PSBequivalent=0
  Current Measurement5 : spsCurrentMeasurementLib/Current Measurement  PhasorSimulation=off  OutputType=Complex  PSBequivalent=0
  DC Voltage Source : spsDCVoltageSourceLib/DC Voltage Source  Amplitude=100  Measurements=None
  DocBlock : simulink/Model-Wide Utilities/DocBlock  DocumentType=Text
      content=|
      | Ramp is added to reference to avoid subharmonic oscilations.
      |
      | Check NxP AN4716: https://www.nxp.com/docs/en/application-note/AN4716.pdf
  Gain : Gain  Gain=-0.1
  Mosfet{,1..3} (4 alike) : spsMosfetLib/Mosfet  Ron=0.1  Lon=0  Rd=0.01  Vfd=0  IC=0  Rs=1e5  Cs=inf  Measurements=off
  PWM : simulink/Discontinuities/PWM  DisableCoverage=on  Period=1E-5  DisallowZeroDutyCycle=off  RunAtFixedTimeIntervals=off  SampleTime=0.1
  Ramp Reference : spsSawtoothGeneratorLib/Sawtooth Generator  Freq=10e3  Phase=0  Ts=0
  Relational Operator : RelationalOperator  OutDataTypeStr=boolean  RndMeth=Simplest
  Scope1 : Scope  NumInputPorts=4
  Scope2 : Scope  NumInputPorts=3
  Series RLC Branch7 : spsSeriesRLCBranchLib/Series RLC Branch  LConnTagsString=__new0  RConnTagsString=__new0  BranchType=L  Resistance=1  Inductance=cfg.main_L  SetiL0=off  InitialCurrent=0  Capacitance=1e-6  Setx0=off  InitialVoltage=0  Measurements=Branch current
  Series RLC Branch8 : spsSeriesRLCBranchLib/Series RLC Branch  LConnTagsString=__new0  RConnTagsString=__new0  BranchType=L  Resistance=1  Inductance=cfg.main_L  SetiL0=off  InitialCurrent=0  Capacitance=1e-6  Setx0=off  InitialVoltage=0  Measurements=Branch current
  Set-Reset Flip-Flop : eeGeneralControl/Set-Reset Flip-Flop  LabelModeActiveChoice=Discrete  UndefState=Reset  Q0=0  Ts=-1
      settings: SourceProductBaseCode=PS
  powergui1 : spspowerguiLib/powergui  Priority=1  SimulationMode=Discrete  SampleTime=1e-8  frequency=60  Iterations=50  frequencyindice=0  Pbase=100e6  ErrMax=1e-4  UnitsV=kV  UnitsW=MW  buscounter=0  FunctionMessages=off  echomessages=off  EnableUseOfTLC=off  CurrentSourceSwitches=off  DisableSnubberDevices=off  DisableRonSwitches=off  DisableVfSwitches=off  DisplayEquations=off  AutomaticDiscreteSolvers=off  SolverType=Tustin/Backward Euler (TBE)  Interpol=off  ExternalGateDelay=off  methode=off  Ts=100  x0status=blocks  SPID=on  SwTol=0  HookPort=off  NonlinearTolerance=1e-4  nMaxIteration=100  ContinueOnMaxIteration=off  RestoreLinks=warning  ResistiveCurrentMeasurement=off  Frange=[0:2:500]  Ylog=off  Xlog=on  ShowGrid=off  save=off  variable=ZData  structure=0  ZoomFFT=off  StartTime=0.0  cycles=1  DisplayStyle=1  fundamental=60  FreqAxis=off  MaxFrequency=1000  frequencyindicesteady=1  RmsSteady=1  display=off
  Connection Port1 : PMIOPort  Side=Right
  Connection Port : PMIOPort  Port=2  Side=Right
  wires:
  Current Measurement5/1 -> [I_source]
  [gate_2] -> Mosfet/1
  Current Measurement4/1 -> Scope2/3, Add2/2
  PWM/1 -> Set-Reset Flip-Flop/2, Scope1/3
  Set-Reset Flip-Flop/1 -> [gate_2]
  Ramp Reference/1 -> Gain/1
  [gate_1] -> Scope1/2
  [I_source] -> Scope2/1
  Constant4/1 -> Mosfet3/1
  Add2/1 -> Relational Operator/2
  Constant2/1 -> PWM/1
  Constant3/1 -> Mosfet2/1
  Add1/1 -> Scope2/2, Add2/1
  [gate_1] -> Mosfet1/1
  Gain/1 -> Add1/1
  Input/1 -> Add1/2
  [gate_2] -> Scope1/1
  Set-Reset Flip-Flop/2 -> [gate_1]
  Relational Operator/1 -> Set-Reset Flip-Flop/1, Scope1/4
  Constant1/1 -> Relational Operator/1
  connections:
  Mosfet2/LConn1 -- Mosfet/LConn1 -- Current Measurement5/RConn1
  Series RLC Branch7/RConn1 -- Connection Port/RConn1
  Mosfet3/RConn1 -- Mosfet1/RConn1 -- DC Voltage Source/LConn1
  Current Measurement4/LConn1 -- Series RLC Branch7/LConn1
  Connection Port1/RConn1 -- Series RLC Branch8/RConn1
  Current Measurement5/LConn1 -- DC Voltage Source/RConn1
  Current Measurement4/RConn1 -- Mosfet1/LConn1 -- Mosfet/RConn1
  Mosfet2/RConn1 -- Series RLC Branch8/LConn1 -- Mosfet3/LConn1

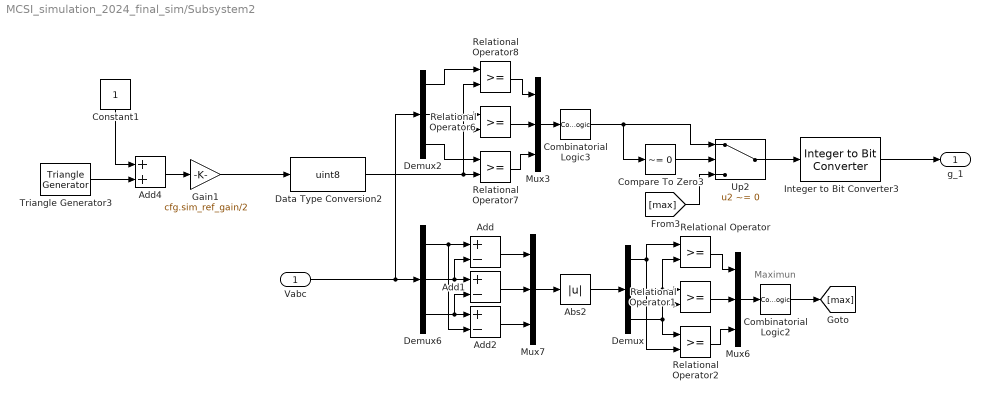
== system MCSI_simulation_2024_final_sim/Subsystem2 ==
  note: Maximun
  Vabc : Inport
  Abs2 : Abs
  Add : Sum  Inputs=+-
  Add1 : Sum  Inputs=+-
  Add2 : Sum  Inputs=+-
  Add4 : Sum
  Combinatorial Logic2 : CombinatorialLogic  TruthTable=bin2dec(['111111'; '001001'; '010010'; '010010'; '100100'; '001001'; '100100'; '111111'])
  Combinatorial Logic3 : CombinatorialLogic  TruthTable=bin2dec(['000000'; '001010'; '010100'; '001100'; '100001'; '100010'; '010001'; '000000'])
  Compare To Zero3 : simulink/Logic and Bit Operations/Compare To Zero  relop=~=  OutDataTypeStr=boolean
  Constant1 : Constant
  Data Type Conversion2 : DataTypeConversion  OutDataTypeStr=uint8
  Demux : Demux  Outputs=3
  Demux2 : Demux  Outputs=3
  Demux6 : Demux  Outputs=3
  Gain1 : Gain  Gain=cfg.sim_ref_gain/2
  Integer to Bit Converter3 : commutil2/Integer to Bit Converter  nbits=6  signedInputValues=Unsigned  bitOrder=MSB first  outDtype=Inherit via internal rule
  Mux3 : Mux  Inputs=3
  Mux6 : Mux  Inputs=3
  Mux7 : Mux  Inputs=3
  Relational Operator{,1..2,6..8} (6 alike) : RelationalOperator  OutDataTypeStr=boolean  RndMeth=Nearest
  Triangle Generator3 : spsTriangleGeneratorLib/Triangle Generator  Freq=cfg.fl*cfg.mf  Phase=0  Ts=cfg.ts
  Up2 : Switch  Criteria=u2 ~= 0
  g_1 : Outport
  wires:
  Relational Operator/1 -> Mux6/1
  Demux/3 -> Relational Operator1/2, Relational Operator2/1
  Relational Operator1/1 -> Mux6/2
  Demux/2 -> Relational Operator/2, Relational Operator1/1
  Mux6/1 -> Combinatorial Logic2/1
  Relational Operator2/1 -> Mux6/3
  Demux/1 -> Relational Operator/1, Relational Operator2/2
  Demux6/1 -> Add2/2, Add/1
  Demux6/2 -> Add/2, Add1/1
  Demux6/3 -> Add1/2, Add2/1
  Add/1 -> Mux7/1
  Add1/1 -> Mux7/2
  Add2/1 -> Mux7/3
  Abs2/1 -> Demux/1
  Mux7/1 -> Abs2/1
  Combinatorial Logic2/1 -> [max]
  Relational Operator7/1 -> Mux3/3
  Relational Operator8/1 -> Mux3/1
  Relational Operator6/1 -> Mux3/2
  Mux3/1 -> Combinatorial Logic3/1
  Combinatorial Logic3/1 -> Up2/1, Compare To Zero3/1
  Compare To Zero3/1 -> Up2/2
  Up2/1 -> Integer to Bit Converter3/1
  [max] -> Up2/3
  Demux2/3 -> Relational Operator7/1
  Demux2/2 -> Relational Operator6/1
  Demux2/1 -> Relational Operator8/1
  Integer to Bit Converter3/1 -> g_1/1
  Vabc/1 -> Demux2/1, Demux6/1
  Data Type Conversion2/1 -> Relational Operator8/2, Relational Operator6/2, Relational Operator7/2
  Gain1/1 -> Data Type Conversion2/1
  ? -> ?
  Constant1/1 -> Add4/1
  Triangle Generator3/1 -> Add4/2
  Add4/1 -> Gain1/1

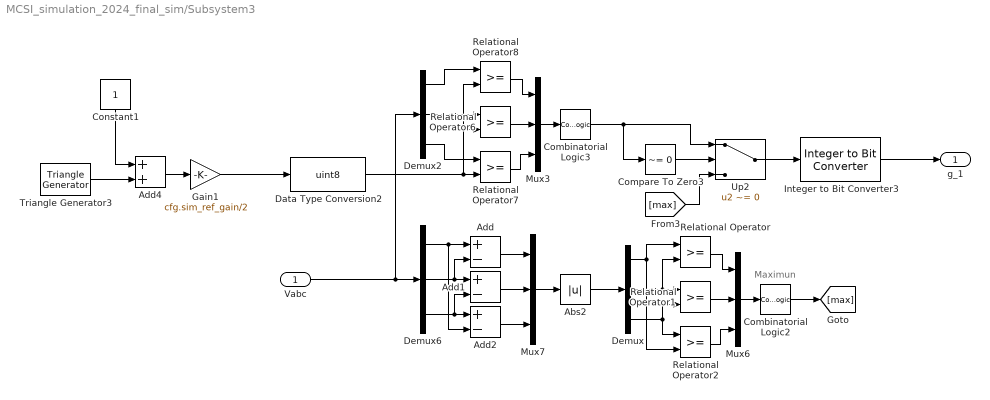
== system MCSI_simulation_2024_final_sim/Subsystem3 ==
  note: Maximun
  Vabc : Inport
  Abs2 : Abs
  Add : Sum  Inputs=+-
  Add1 : Sum  Inputs=+-
  Add2 : Sum  Inputs=+-
  Add4 : Sum
  Combinatorial Logic2 : CombinatorialLogic  TruthTable=bin2dec(['111111'; '001001'; '010010'; '010010'; '100100'; '001001'; '100100'; '111111'])
  Combinatorial Logic3 : CombinatorialLogic  TruthTable=bin2dec(['000000'; '001010'; '010100'; '001100'; '100001'; '100010'; '010001'; '000000'])
  Compare To Zero3 : simulink/Logic and Bit Operations/Compare To Zero  relop=~=  OutDataTypeStr=boolean
  Constant1 : Constant
  Data Type Conversion2 : DataTypeConversion  OutDataTypeStr=uint8
  Demux : Demux  Outputs=3
  Demux2 : Demux  Outputs=3
  Demux6 : Demux  Outputs=3
  Gain1 : Gain  Gain=cfg.sim_ref_gain/2
  Integer to Bit Converter3 : commutil2/Integer to Bit Converter  nbits=6  signedInputValues=Unsigned  bitOrder=MSB first  outDtype=Inherit via internal rule
  Mux3 : Mux  Inputs=3
  Mux6 : Mux  Inputs=3
  Mux7 : Mux  Inputs=3
  Relational Operator{,1..2,6..8} (6 alike) : RelationalOperator  OutDataTypeStr=boolean  RndMeth=Nearest
  Triangle Generator3 : spsTriangleGeneratorLib/Triangle Generator  Freq=cfg.fl*cfg.mf  Phase=0  Ts=cfg.ts
  Up2 : Switch  Criteria=u2 ~= 0
  g_1 : Outport
  wires:
  Relational Operator/1 -> Mux6/1
  Demux/3 -> Relational Operator1/2, Relational Operator2/1
  Relational Operator1/1 -> Mux6/2
  Demux/2 -> Relational Operator/2, Relational Operator1/1
  Mux6/1 -> Combinatorial Logic2/1
  Relational Operator2/1 -> Mux6/3
  Demux/1 -> Relational Operator/1, Relational Operator2/2
  Demux6/1 -> Add2/2, Add/1
  Demux6/2 -> Add/2, Add1/1
  Demux6/3 -> Add1/2, Add2/1
  Add/1 -> Mux7/1
  Add1/1 -> Mux7/2
  Add2/1 -> Mux7/3
  Abs2/1 -> Demux/1
  Mux7/1 -> Abs2/1
  Combinatorial Logic2/1 -> [max]
  Relational Operator7/1 -> Mux3/3
  Relational Operator8/1 -> Mux3/1
  Relational Operator6/1 -> Mux3/2
  Mux3/1 -> Combinatorial Logic3/1
  Combinatorial Logic3/1 -> Up2/1, Compare To Zero3/1
  Compare To Zero3/1 -> Up2/2
  Up2/1 -> Integer to Bit Converter3/1
  [max] -> Up2/3
  Demux2/3 -> Relational Operator7/1
  Demux2/2 -> Relational Operator6/1
  Demux2/1 -> Relational Operator8/1
  Integer to Bit Converter3/1 -> g_1/1
  Vabc/1 -> Demux2/1, Demux6/1
  Data Type Conversion2/1 -> Relational Operator8/2, Relational Operator6/2, Relational Operator7/2
  Gain1/1 -> Data Type Conversion2/1
  ? -> ?
  Constant1/1 -> Add4/1
  Triangle Generator3/1 -> Add4/2
  Add4/1 -> Gain1/1

== system MCSI_simulation_2024_final_sim/SPWM_3mod_hdl/Maximum Calculator ==
  3 phase Vab0 : Inport
  3 phase Vab120 : Inport  Port=2
  3 phase Vab240 : Inport  Port=3
  Abs : Abs
  Abs1 : Abs
  Abs2 : Abs
  Bit Concat : hdlsllib/Logic and Bit Operations/Bit Concat  numInputs=6
  Decoder : Subsystem
  Logical Operator{,1..5} (6 alike) : Logic  Operator=OR  Inputs=4  IconShape=distinctive  AllPortsSameDT=off  OutDataTypeStr=boolean
  Relational Operator : RelationalOperator  OutDataTypeStr=boolean  RndMeth=Nearest
  Relational Operator1 : RelationalOperator  OutDataTypeStr=boolean  RndMeth=Nearest
  Relational Operator2 : RelationalOperator  OutDataTypeStr=boolean  RndMeth=Nearest
  Subtract : Sum  Inputs=+-  OutDataTypeStr=int16
  Subtract1 : Sum  Inputs=+-  OutDataTypeStr=int16
  Subtract2 : Sum  Inputs=+-  OutDataTypeStr=int16
  g_max : Outport  VectorParamsAs1DForOutWhenUnconnected=off
  wires:
  Relational Operator/1 -> Decoder/1(b2)
  Abs1/1 -> Relational Operator/1, Relational Operator2/2
  Logical Operator2/1 -> Bit Concat/3
  Abs/1 -> Relational Operator/2, Relational Operator1/1
  3 phase Vab0/1 -> Subtract2/2, Subtract/1
  Decoder/6(Out6) -> Logical Operator5/3, Logical Operator2/3
  Decoder/3(Out3) -> Logical Operator4/2, Logical Operator1/2
  Decoder/2(Out2) -> Logical Operator2/2, Logical Operator5/2
  3 phase Vab240/1 -> Subtract2/1, Subtract1/2
  Logical Operator5/1 -> Bit Concat/6
  Decoder/1(Out1) -> Logical Operator1/1, Logical Operator/1, Logical Operator5/1, Logical Operator4/1, Logical Operator3/1, Logical Operator2/1
  Abs2/1 -> Relational Operator1/2, Relational Operator2/1
  Subtract1/1 -> Abs/1
  Decoder/4(Out4) -> Logical Operator4/3, Logical Operator1/3
  3 phase Vab120/1 -> Subtract1/1, Subtract/2
  Logical Operator3/1 -> Bit Concat/4
  Decoder/5(Out5) -> Logical Operator3/2, Logical Operator/2
  Subtract/1 -> Abs1/1
  Subtract2/1 -> Abs2/1
  Relational Operator1/1 -> Decoder/2(b1)
  Relational Operator2/1 -> Decoder/3(b0 (LSB))
  Logical Operator1/1 -> Bit Concat/2
  Decoder/8(Out8) -> Logical Operator/4, Logical Operator1/4, Logical Operator2/4, Logical Operator3/4, Logical Operator4/4, Logical Operator5/4
  Decoder/7(Out7) -> Logical Operator3/3, Logical Operator/3
  Logical Operator4/1 -> Bit Concat/5
  Logical Operator/1 -> Bit Concat/1
  Bit Concat/1 -> g_max/1

== system MCSI_simulation_2024_final_sim/SPWM_3mod_hdl/tabla_spwm_g1 ==
  In2 : Inport
  In3 : Inport  Port=2
  In4 : Inport  Port=3
  Bit Concat : hdlsllib/Logic and Bit Operations/Bit Concat  numInputs=6
  Decoder : Subsystem
  Logical Operator{,1,4..7} (6 alike) : Logic  Operator=OR  IconShape=distinctive  AllPortsSameDT=off  OutDataTypeStr=boolean
  Terminator : Terminator
  Terminator1 : Terminator
  g_out : Outport  VectorParamsAs1DForOutWhenUnconnected=off
  wires:
  Decoder/7(Out7) -> Logical Operator1/2, Logical Operator7/2
  Logical Operator4/1 -> Bit Concat/3
  Logical Operator/1 -> Bit Concat/1
  Logical Operator1/1 -> Bit Concat/2
  Decoder/2(Out2) -> Logical Operator4/1, Logical Operator6/1
  Logical Operator7/1 -> Bit Concat/6
  Logical Operator5/1 -> Bit Concat/4
  Decoder/5(Out5) -> Logical Operator/1, Logical Operator7/1
  Logical Operator6/1 -> Bit Concat/5
  In4/1 -> Decoder/3(b0 (LSB))
  In3/1 -> Decoder/2(b1)
  In2/1 -> Decoder/1(b2)
  Decoder/4(Out4) -> Logical Operator5/2, Logical Operator4/2
  Decoder/3(Out3) -> Logical Operator5/1, Logical Operator1/1
  Decoder/6(Out6) -> Logical Operator/2, Logical Operator6/2
  Decoder/1(Out1) -> Terminator/1
  Decoder/8(Out8) -> Terminator1/1
  Bit Concat/1 -> g_out/1

== system MCSI_simulation_2024_final_sim/SPWM_3mod_hdl1/Maximum Calculator ==
  3 phase Vab0 : Inport
  3 phase Vab120 : Inport  Port=2
  3 phase Vab240 : Inport  Port=3
  Abs : Abs
  Abs1 : Abs
  Abs2 : Abs
  Bit Concat : hdlsllib/Logic and Bit Operations/Bit Concat  numInputs=6
  Decoder : Subsystem
  Logical Operator{,1..5} (6 alike) : Logic  Operator=OR  Inputs=4  IconShape=distinctive  AllPortsSameDT=off  OutDataTypeStr=boolean
  Relational Operator : RelationalOperator  OutDataTypeStr=boolean  RndMeth=Nearest
  Relational Operator1 : RelationalOperator  OutDataTypeStr=boolean  RndMeth=Nearest
  Relational Operator2 : RelationalOperator  OutDataTypeStr=boolean  RndMeth=Nearest
  Subtract : Sum  Inputs=+-  OutDataTypeStr=int16
  Subtract1 : Sum  Inputs=+-  OutDataTypeStr=int16
  Subtract2 : Sum  Inputs=+-  OutDataTypeStr=int16
  g_max : Outport  VectorParamsAs1DForOutWhenUnconnected=off
  wires:
  Relational Operator/1 -> Decoder/1(b2)
  Abs1/1 -> Relational Operator/1, Relational Operator2/2
  Logical Operator2/1 -> Bit Concat/3
  Abs/1 -> Relational Operator/2, Relational Operator1/1
  3 phase Vab0/1 -> Subtract2/2, Subtract/1
  Decoder/6(Out6) -> Logical Operator5/3, Logical Operator2/3
  Decoder/3(Out3) -> Logical Operator4/2, Logical Operator1/2
  Decoder/2(Out2) -> Logical Operator2/2, Logical Operator5/2
  3 phase Vab240/1 -> Subtract2/1, Subtract1/2
  Logical Operator5/1 -> Bit Concat/6
  Decoder/1(Out1) -> Logical Operator1/1, Logical Operator/1, Logical Operator5/1, Logical Operator4/1, Logical Operator3/1, Logical Operator2/1
  Abs2/1 -> Relational Operator1/2, Relational Operator2/1
  Subtract1/1 -> Abs/1
  Decoder/4(Out4) -> Logical Operator4/3, Logical Operator1/3
  3 phase Vab120/1 -> Subtract1/1, Subtract/2
  Logical Operator3/1 -> Bit Concat/4
  Decoder/5(Out5) -> Logical Operator3/2, Logical Operator/2
  Subtract/1 -> Abs1/1
  Subtract2/1 -> Abs2/1
  Relational Operator1/1 -> Decoder/2(b1)
  Relational Operator2/1 -> Decoder/3(b0 (LSB))
  Logical Operator1/1 -> Bit Concat/2
  Decoder/8(Out8) -> Logical Operator/4, Logical Operator1/4, Logical Operator2/4, Logical Operator3/4, Logical Operator4/4, Logical Operator5/4
  Decoder/7(Out7) -> Logical Operator3/3, Logical Operator/3
  Logical Operator4/1 -> Bit Concat/5
  Logical Operator/1 -> Bit Concat/1
  Bit Concat/1 -> g_max/1

== system MCSI_simulation_2024_final_sim/SPWM_3mod_hdl1/tabla_spwm_g1 ==
  In2 : Inport
  In3 : Inport  Port=2
  In4 : Inport  Port=3
  Bit Concat : hdlsllib/Logic and Bit Operations/Bit Concat  numInputs=6
  Decoder : Subsystem
  Logical Operator{,1,4..7} (6 alike) : Logic  Operator=OR  IconShape=distinctive  AllPortsSameDT=off  OutDataTypeStr=boolean
  Terminator : Terminator
  Terminator1 : Terminator
  g_out : Outport  VectorParamsAs1DForOutWhenUnconnected=off
  wires:
  Decoder/7(Out7) -> Logical Operator1/2, Logical Operator7/2
  Logical Operator4/1 -> Bit Concat/3
  Logical Operator/1 -> Bit Concat/1
  Logical Operator1/1 -> Bit Concat/2
  Decoder/2(Out2) -> Logical Operator4/1, Logical Operator6/1
  Logical Operator7/1 -> Bit Concat/6
  Logical Operator5/1 -> Bit Concat/4
  Decoder/5(Out5) -> Logical Operator/1, Logical Operator7/1
  Logical Operator6/1 -> Bit Concat/5
  In4/1 -> Decoder/3(b0 (LSB))
  In3/1 -> Decoder/2(b1)
  In2/1 -> Decoder/1(b2)
  Decoder/4(Out4) -> Logical Operator5/2, Logical Operator4/2
  Decoder/3(Out3) -> Logical Operator5/1, Logical Operator1/1
  Decoder/6(Out6) -> Logical Operator/2, Logical Operator6/2
  Decoder/1(Out1) -> Terminator/1
  Decoder/8(Out8) -> Terminator1/1
  Bit Concat/1 -> g_out/1

== system MCSI_simulation_2024_final_sim/SPWM_3mod_hdl2/Maximum Calculator ==
  3 phase Vab0 : Inport
  3 phase Vab120 : Inport  Port=2
  3 phase Vab240 : Inport  Port=3
  Abs : Abs
  Abs1 : Abs
  Abs2 : Abs
  Bit Concat : hdlsllib/Logic and Bit Operations/Bit Concat  numInputs=6
  Decoder : Subsystem
  Logical Operator{,1..5} (6 alike) : Logic  Operator=OR  Inputs=4  IconShape=distinctive  AllPortsSameDT=off  OutDataTypeStr=boolean
  Relational Operator : RelationalOperator  OutDataTypeStr=boolean  RndMeth=Nearest
  Relational Operator1 : RelationalOperator  OutDataTypeStr=boolean  RndMeth=Nearest
  Relational Operator2 : RelationalOperator  OutDataTypeStr=boolean  RndMeth=Nearest
  Subtract : Sum  Inputs=+-  OutDataTypeStr=int16
  Subtract1 : Sum  Inputs=+-  OutDataTypeStr=int16
  Subtract2 : Sum  Inputs=+-  OutDataTypeStr=int16
  g_max : Outport  VectorParamsAs1DForOutWhenUnconnected=off
  wires:
  Relational Operator/1 -> Decoder/1(b2)
  Abs1/1 -> Relational Operator/1, Relational Operator2/2
  Logical Operator2/1 -> Bit Concat/3
  Abs/1 -> Relational Operator/2, Relational Operator1/1
  3 phase Vab0/1 -> Subtract2/2, Subtract/1
  Decoder/6(Out6) -> Logical Operator5/3, Logical Operator2/3
  Decoder/3(Out3) -> Logical Operator4/2, Logical Operator1/2
  Decoder/2(Out2) -> Logical Operator2/2, Logical Operator5/2
  3 phase Vab240/1 -> Subtract2/1, Subtract1/2
  Logical Operator5/1 -> Bit Concat/6
  Decoder/1(Out1) -> Logical Operator1/1, Logical Operator/1, Logical Operator5/1, Logical Operator4/1, Logical Operator3/1, Logical Operator2/1
  Abs2/1 -> Relational Operator1/2, Relational Operator2/1
  Subtract1/1 -> Abs/1
  Decoder/4(Out4) -> Logical Operator4/3, Logical Operator1/3
  3 phase Vab120/1 -> Subtract1/1, Subtract/2
  Logical Operator3/1 -> Bit Concat/4
  Decoder/5(Out5) -> Logical Operator3/2, Logical Operator/2
  Subtract/1 -> Abs1/1
  Subtract2/1 -> Abs2/1
  Relational Operator1/1 -> Decoder/2(b1)
  Relational Operator2/1 -> Decoder/3(b0 (LSB))
  Logical Operator1/1 -> Bit Concat/2
  Decoder/8(Out8) -> Logical Operator/4, Logical Operator1/4, Logical Operator2/4, Logical Operator3/4, Logical Operator4/4, Logical Operator5/4
  Decoder/7(Out7) -> Logical Operator3/3, Logical Operator/3
  Logical Operator4/1 -> Bit Concat/5
  Logical Operator/1 -> Bit Concat/1
  Bit Concat/1 -> g_max/1

== system MCSI_simulation_2024_final_sim/SPWM_3mod_hdl2/tabla_spwm_g1 ==
  In2 : Inport
  In3 : Inport  Port=2
  In4 : Inport  Port=3
  Bit Concat : hdlsllib/Logic and Bit Operations/Bit Concat  numInputs=6
  Decoder : Subsystem
  Logical Operator{,1,4..7} (6 alike) : Logic  Operator=OR  IconShape=distinctive  AllPortsSameDT=off  OutDataTypeStr=boolean
  Terminator : Terminator
  Terminator1 : Terminator
  g_out : Outport  VectorParamsAs1DForOutWhenUnconnected=off
  wires:
  Decoder/7(Out7) -> Logical Operator1/2, Logical Operator7/2
  Logical Operator4/1 -> Bit Concat/3
  Logical Operator/1 -> Bit Concat/1
  Logical Operator1/1 -> Bit Concat/2
  Decoder/2(Out2) -> Logical Operator4/1, Logical Operator6/1
  Logical Operator7/1 -> Bit Concat/6
  Logical Operator5/1 -> Bit Concat/4
  Decoder/5(Out5) -> Logical Operator/1, Logical Operator7/1
  Logical Operator6/1 -> Bit Concat/5
  In4/1 -> Decoder/3(b0 (LSB))
  In3/1 -> Decoder/2(b1)
  In2/1 -> Decoder/1(b2)
  Decoder/4(Out4) -> Logical Operator5/2, Logical Operator4/2
  Decoder/3(Out3) -> Logical Operator5/1, Logical Operator1/1
  Decoder/6(Out6) -> Logical Operator/2, Logical Operator6/2
  Decoder/1(Out1) -> Terminator/1
  Decoder/8(Out8) -> Terminator1/1
  Bit Concat/1 -> g_out/1

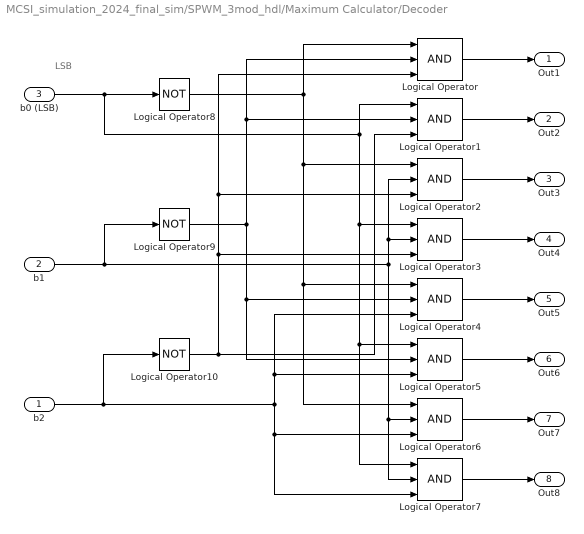
== system MCSI_simulation_2024_final_sim/SPWM_3mod_hdl/Maximum Calculator/Decoder ==
  note: LSB
  b2 : Inport
  b1 : Inport  Port=2
  b0 (LSB) : Inport  Port=3
  Logical Operator{,1..7} (8 alike) : Logic  Inputs=3  IconShape=distinctive  AllPortsSameDT=off  OutDataTypeStr=boolean
  Logical Operator10 : Logic  Operator=NOT  IconShape=distinctive  AllPortsSameDT=off  OutDataTypeStr=boolean
  Logical Operator8 : Logic  Operator=NOT  IconShape=distinctive  AllPortsSameDT=off  OutDataTypeStr=boolean
  Logical Operator9 : Logic  Operator=NOT  IconShape=distinctive  AllPortsSameDT=off  OutDataTypeStr=boolean
  Out1 : Outport
  Out2 : Outport  Port=2
  Out3 : Outport  Port=3
  Out4 : Outport  Port=4
  Out5 : Outport  Port=5
  Out6 : Outport  Port=6
  Out7 : Outport  Port=7
  Out8 : Outport  Port=8
  wires:
  Logical Operator9/1 -> Logical Operator5/2, Logical Operator4/2, Logical Operator1/2, Logical Operator/2
  Logical Operator5/1 -> Out6/1
  Logical Operator1/1 -> Out2/1
  Logical Operator10/1 -> Logical Operator3/3, Logical Operator2/3, Logical Operator/3, Logical Operator1/3
  Logical Operator/1 -> Out1/1
  Logical Operator8/1 -> Logical Operator6/1, Logical Operator4/1, Logical Operator2/1, Logical Operator/1
  b2/1 -> Logical Operator4/3, Logical Operator5/3, Logical Operator7/3, Logical Operator6/3, Logical Operator10/1
  b0 (LSB)/1 -> Logical Operator7/1, Logical Operator5/1, Logical Operator3/1, Logical Operator1/1, Logical Operator8/1
  Logical Operator7/1 -> Out8/1
  b1/1 -> Logical Operator3/2, Logical Operator2/2, Logical Operator7/2, Logical Operator6/2, Logical Operator9/1
  Logical Operator4/1 -> Out5/1
  Logical Operator6/1 -> Out7/1
  Logical Operator3/1 -> Out4/1
  Logical Operator2/1 -> Out3/1
